simulink model "solar_tracker_SIL_controller"  (R2025b)
settings: Solver=ode4  StartTime=0  StopTime=60  FixedStep=0.01  RelTol=1e-3
settings Model: Creator=Kerem Bayer  LastModifiedBy=Kerem Bayer

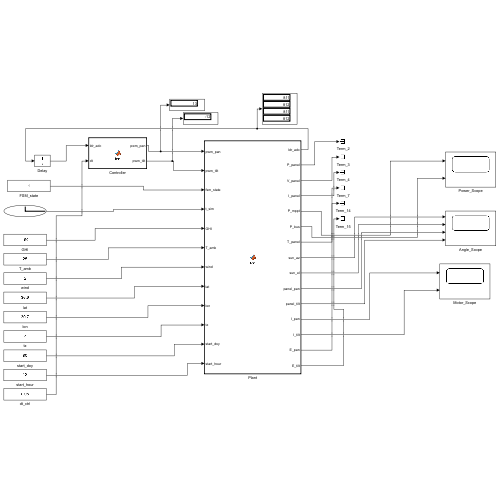
[thumbnail: Simulink's stored preview of the top-level diagram]
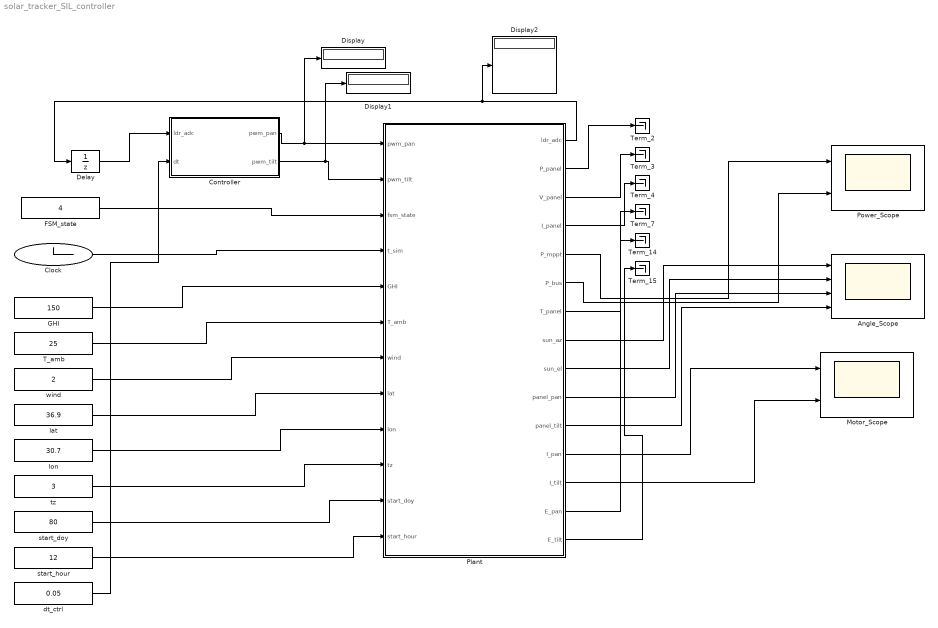
== system solar_tracker_SIL_controller ==
  Angle_Scope : Scope  NumInputPorts=4
      settings: ActiveDisplayYMinimum=-67.998723649447911  ActiveDisplayYMaximum=173.56640204477748
  Clock : Clock
  Controller : MATLAB Function  TreatAsAtomicUnit=on
  Delay : UnitDelay  InitialCondition=zeros(1,4,'uint16')  SampleTime=-1  HasFrameUpgradeWarning=on
  Display : Display
  Display1 : Display
  Display2 : Display
  FSM_state : Constant  Value=4  OutDataTypeStr=uint8
  GHI : Constant  Value=150  OutDataTypeStr=double
  Motor_Scope : Scope  NumInputPorts=2
      settings: ActiveDisplayYMinimum=-0.15193498150664253  ActiveDisplayYMaximum=1.2889406434933575
  Plant : MATLAB Function  TreatAsAtomicUnit=on
  Power_Scope : Scope  NumInputPorts=2
      settings: ActiveDisplayYMinimum=-1  ActiveDisplayYMaximum=1
  T_amb : Constant  Value=25  OutDataTypeStr=double
  Term_{2..4,7,14..15} (6 alike) : Terminator
  dt_ctrl : Constant  Value=0.05  OutDataTypeStr=double
  lat : Constant  Value=36.9  OutDataTypeStr=double
  lon : Constant  Value=30.7  OutDataTypeStr=double
  start_doy : Constant  Value=80  OutDataTypeStr=double
  start_hour : Constant  Value=12  OutDataTypeStr=double
  tz : Constant  Value=3  OutDataTypeStr=double
  wind : Constant  Value=2  OutDataTypeStr=double
  wires:
  Plant/1(ldr_adc) -> Display2/1, Delay/1
  Delay/1 -> Controller/1(ldr_adc)
  dt_ctrl/1 -> Controller/2(dt)
  Controller/1(pwm_pan) -> Plant/1(pwm_pan), Display/1
  Controller/2(pwm_tilt) -> Display1/1, Plant/2(pwm_tilt)
  FSM_state/1 -> Plant/3(fsm_state)
  Clock/1 -> Plant/4(t_sim)
  GHI/1 -> Plant/5(GHI)
  T_amb/1 -> Plant/6(T_amb)
  wind/1 -> Plant/7(wind)
  lat/1 -> Plant/8(lat)
  lon/1 -> Plant/9(lon)
  tz/1 -> Plant/10(tz)
  start_doy/1 -> Plant/11(start_doy)
  start_hour/1 -> Plant/12(start_hour)
  Plant/5(P_mppt) -> Power_Scope/1
  Plant/6(P_bus) -> Power_Scope/2
  Plant/8(sun_az) -> Angle_Scope/1
  Plant/9(sun_el) -> Angle_Scope/2
  Plant/10(panel_pan) -> Angle_Scope/3
  Plant/11(panel_tilt) -> Angle_Scope/4
  Plant/12(I_pan) -> Motor_Scope/1
  Plant/13(I_tilt) -> Motor_Scope/2
  Plant/2(P_panel) -> Term_2/1
  Plant/3(V_panel) -> Term_3/1
  Plant/4(I_panel) -> Term_4/1
  Plant/7(T_panel) -> Term_7/1
  Plant/14(E_pan) -> Term_14/1
  Plant/15(E_tilt) -> Term_15/1

== matlab function solar_tracker_SIL_controller/Plant ==
  data: pwm_pan input; ldr_adc output; pwm_tilt input; fsm_state input; t_sim input; GHI input; T_amb input; wind input; lat input; lon input; tz input; start_doy input; start_hour input; P_panel output; V_panel output; I_panel output; P_mppt output; P_bus output; T_panel output; sun_az output; sun_el output; panel_pan output; panel_tilt output; I_pan output; I_tilt output; E_pan output; E_tilt output
function [ldr_adc, P_panel, V_panel, I_panel, P_mppt, P_bus, ...
          T_panel, sun_az, sun_el, panel_pan, panel_tilt, ...
          I_pan, I_tilt, E_pan, E_tilt] = fcn( ...
          pwm_pan, pwm_tilt, fsm_state, t_sim, GHI, T_amb, wind, ...
          lat, lon, tz, start_doy, start_hour)
    coder.extrinsic('plant_step');

    ldr_adc    = uint16(zeros(1,4));
    P_panel    = zeros(4,1);
    V_panel    = zeros(4,1);
    I_panel    = zeros(4,1);
    T_panel    = zeros(4,1);
    P_mppt     = 0;   P_bus = 0;
    sun_az     = 0;   sun_el = 0;
    panel_pan  = 0;   panel_tilt = 0;
    I_pan      = 0;   I_tilt = 0;
    E_pan      = 0;   E_tilt = 0;

    [ldr_adc, P_panel, V_panel, I_panel, P_mppt, P_bus, ...
     T_panel, sun_az, sun_el, panel_pan, panel_tilt, ...
     I_pan, I_tilt, E_pan, E_tilt] = ...
         plant_step(pwm_pan, pwm_tilt, fsm_state, t_sim, ...
                    GHI, T_amb, wind, ...
                    lat, lon, tz, start_doy, start_hour);
end

== matlab function solar_tracker_SIL_controller/Controller ==
  data: ldr_adc input; pwm_pan output; dt input; pwm_tilt output
function [pwm_pan, pwm_tilt] = fcn(ldr_adc, dt)
    [pwm_pan, pwm_tilt] = controller_step(ldr_adc, dt);
end
